simulink model "last_test2"  (Simulink 7.1)
settings: Solver=ode3  StartTime=0.0  StopTime=2000  FixedStep=0.1  RelTol=1e-3
undefined symbols (not defined in the file or in its folder): C_calc, kalmanfilter4
libraries: fordypningsprosjekt x5, marine_gnc x3, simulink x1
settings Model: Creator=anderga  LastModifiedBy=anders
settings OptimizationCC: SimCompilerOptimization=On

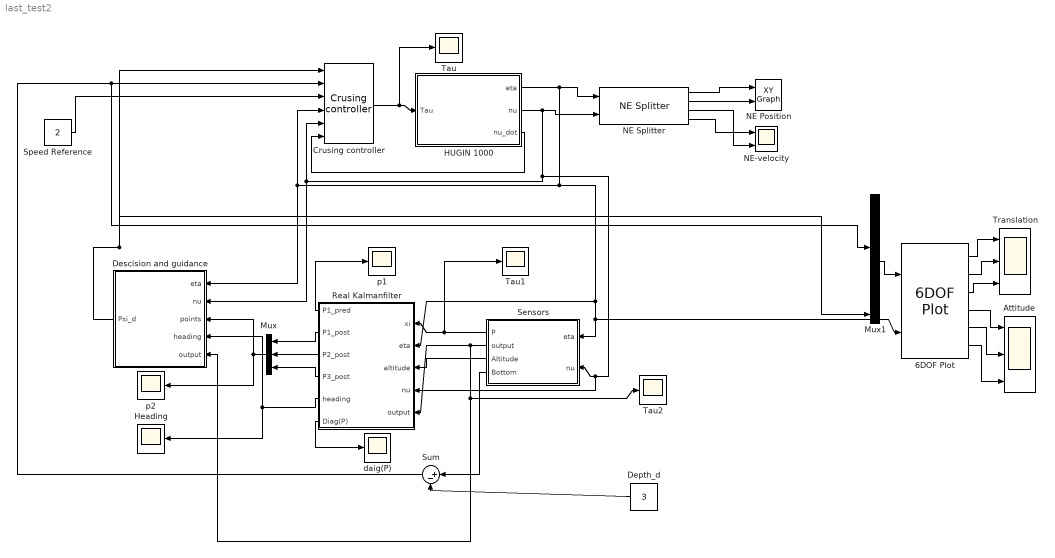
== system last_test2 ==
  6DOF Plot : fordypningsprosjekt/6DOF Plot  SystemSampleTime=-1
  Attitude : Scope  NumInputPorts=3
      settings: TimeRange=700  YMin=-2.5~-10~-50  YMax=2~1~350  SaveName=Attitude
  Crusing controller : fordypningsprosjekt/Crusing controller  SystemSampleTime=-1  Kp_u=10  Ki_u=3  Kp_c=100  Kd_c=100  Kp_d=50  Kp2_d=20  Kd_d=20
  Depth_d : Constant  Orientation=left  Value=3  OutDataType=sfix(16)  OutScaling=2^0
  Descision and guidance : Subsystem  Orientation=left  AncestorBlock=fordypningsprosjekt/Look-ahead guidance
  HUGIN 1000 : Subsystem  AncestorBlock=fordypningsprosjekt/HUGIN 1000  mask(HUGIN 1000 AUV){eta_0=[-30 -30 0 0 0 0], nu_0=[0 0 0 0 0 0], c_on_off=on, beta_c=-45, V_c=0.3}
      mask prompts: eta_0 "Initial Position [x y z phi theta psi]"; nu_0 "Initial speed [u v w p q r]"; c_on_off "Current on"; beta_c "Current heading(deg)"; V_c "Current Velocity"
      mask help:
      | The hydrodynamic model of Kongsberg Maritimes
      | AUV type HUGIN 1000.
      |
      | Implemented using
      |
      | eta_dot = J(eta)*nu
      | M*nu_dot + C(nu)*nu + D(nu)*nu + g(eta) = tau
      |
      | and the MMS toolbox from www.marinecybernetics.org
      mask init:
      | m = 1380;
      | xg = 0;
      | yg = 0;
      | zg = 0.0328;
      | Ix = 86.53;
      | Iy = 1247;
      | Iz = 1247;
      | 
      | Xu = -85.57;
      | Yv = -1092.9;
      | Yr = -84.1448;
      | Zw = -1092.9;
      | Zq = 84.1448;
      | Mq = -795.1686;
      | Nr = -795.1686;
      |     
      | M = [m-Xu   0       0       0       m*zg    -m*yg;
      |      0      m-Yv    0       -m*zg   0       m*xg-Yr;
      |      0      0       m-Zw    m*yg    -m*xg-Zq 0;
      |      0      -m*zg   m*yg    Ix      0        0;
      |      m*zg   0       -m*xg-Zq 0      Iy-Mq    0;
      |      -m*yg  m*xg-Yr 0       0       0       Iz-Nr];
  Heading : Scope
      settings: YMin=1.3258  YMax=1.32584  SaveName=Pipeline_heading
  Mux : Mux  Orientation=left  Inputs=3
  Mux1 : Mux  Inputs=6
  NE Position : simulink/Sinks/XY Graph  SystemSampleTime=-1  xmin=-1000  xmax=1000  ymin=-1000  ymax=1000  st=-1
  NE Splitter : fordypningsprosjekt/NE Splitter  SystemSampleTime=-1
  NE-velocity : Scope  NumInputPorts=2
      settings: YMin=0~-0.25  YMax=2.75~0.2  SaveName=NE_Veloc
  Real Kalmanfilter : Subsystem  Orientation=left  AncestorBlock=fordypningsprosjekt/Real Kalmanfilter
  Sensors : Subsystem  Orientation=left  AncestorBlock=fordypningsprosjekt/Sensors
  Speed Reference : Constant  Value=2  OutDataType=sfix(16)  OutScaling=2^0
  Sum : Sum  Orientation=left  Inputs=|+-  OutDataType=sfix(16)  OutScaling=2^0
  Tau : Scope
      settings: YMin=-3000  YMax=1000  SaveName=Tau_c
  Tau1 : Scope
      settings: TimeRange=700  YMin=-0.5  YMax=0.5  SaveName=Cam_output
  Tau2 : Scope
      settings: TimeRange=700  YMin=0  YMax=1  SaveName=Cam_output1
  Translation : Scope  NumInputPorts=3
      settings: YMin=-150~-200~0  YMax=200~800~12.5  SaveName=Translation
  daig(P) : Scope
      settings: YMin=0  YMax=22.5  SaveName=diag_p_apr
  p1 : Scope
      settings: YMin=0  YMax=500  SaveName=P_pred
  p2 : Scope
      settings: YMin=0  YMax=400  SaveName=P_post
  wires:
  Crusing controller/1 -> HUGIN 1000/1(Tau), Tau/1
  HUGIN 1000/1(eta) -> NE Splitter/1, Real Kalmanfilter/2(eta), Sensors/1(eta), 6DOF Plot/2, Crusing controller/4, Descision and guidance/1(eta)
  HUGIN 1000/2(nu) -> NE Splitter/2, Sensors/2(nu), Real Kalmanfilter/4(nu), Crusing controller/5, Descision and guidance/2(nu)
  NE Splitter/1 -> NE Position/1
  NE Splitter/2 -> NE Position/2
  NE Splitter/4 -> NE-velocity/1
  NE Splitter/3 -> NE-velocity/2
  HUGIN 1000/3(nu_dot) -> Crusing controller/6
  Sensors/1(P) -> Real Kalmanfilter/1(xi), Tau1/1
  Sensors/2(output) -> Descision and guidance/5(output), Tau2/1, Real Kalmanfilter/5(output)
  Sensors/3(Altitude) -> Real Kalmanfilter/3(altitude)
  Depth_d/1 -> Sum/2
  Sensors/4(Bottom) -> Sum/1
  Sum/1 -> Mux1/3, Crusing controller/2
  Speed Reference/1 -> Crusing controller/3
  Descision and guidance/1(Psi_d) -> Mux1/6, Crusing controller/1
  Real Kalmanfilter/5(heading) -> Heading/1, Descision and guidance/4(heading)
  Real Kalmanfilter/2(P1_post) -> Mux/1
  Real Kalmanfilter/3(P2_post) -> Mux/2
  Real Kalmanfilter/4(P3_post) -> Mux/3
  Mux/1 -> p2/1, Descision and guidance/3(points)
  6DOF Plot/1 -> Translation/1
  6DOF Plot/2 -> Translation/2
  6DOF Plot/3 -> Translation/3
  6DOF Plot/4 -> Attitude/1
  6DOF Plot/5 -> Attitude/2
  6DOF Plot/6 -> Attitude/3
  Mux1/1 -> 6DOF Plot/1
  Real Kalmanfilter/1(P1_pred) -> p1/1
  Real Kalmanfilter/6(Diag(P)) -> daig(P)/1

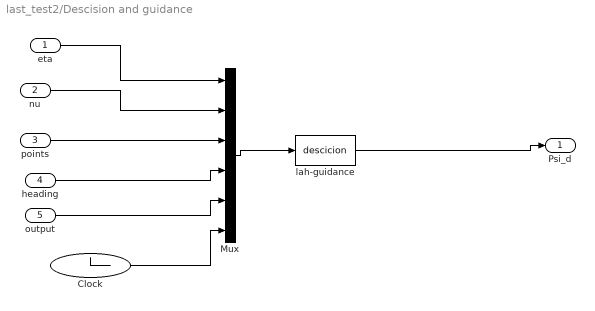
== system last_test2/Descision and guidance ==
  eta : Inport  OutDataType=sfix(16)  OutScaling=2^0
  nu : Inport  Port=2  OutDataType=sfix(16)  OutScaling=2^0
  points : Inport  Port=3  OutDataType=sfix(16)  OutScaling=2^0
  heading : Inport  Port=4  OutDataType=sfix(16)  OutScaling=2^0
  output : Inport  Port=5  OutDataType=sfix(16)  OutScaling=2^0
  Clock : Clock
  Mux : Mux  Inputs=6
  lah-guidance : MATLABFcn  MATLABFcn=descicion  OutputDimensions=1
  Psi_d : Outport  OutDataType=sfix(16)  OutScaling=2^0
  wires:
  heading/1 -> Mux/4
  points/1 -> Mux/3
  eta/1 -> Mux/1
  nu/1 -> Mux/2
  Mux/1 -> lah-guidance/1
  lah-guidance/1 -> Psi_d/1
  output/1 -> Mux/5
  Clock/1 -> Mux/6

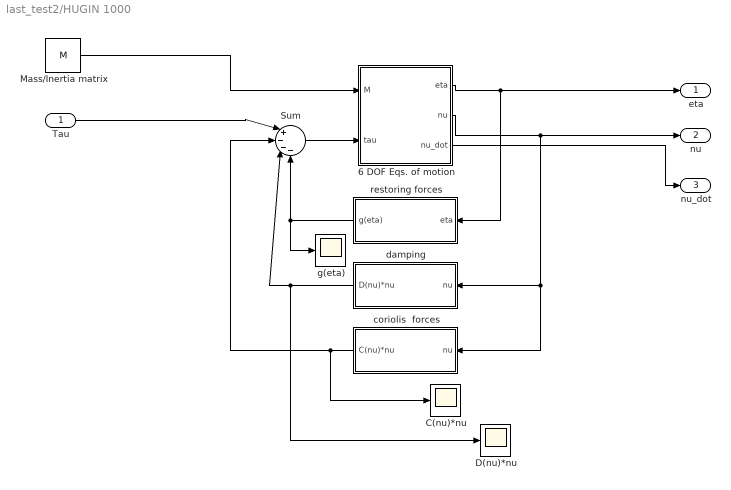
== system last_test2/HUGIN 1000 ==
  Tau : Inport  OutDataType=sfix(16)  OutScaling=2^0
  6 DOF Eqs. of motion : Subsystem  AncestorBlock=marine_gnc/Models/ Kinetics /6 DOF Eqs. of motion  mask(Equations of motion){nu0=nu_0, eta0=eta_0}
      mask prompts: nu0 "Initial velocities (u,v,w,p,q,r)"; eta0 "Initial position/attitude (x,y,z,phi,theta,psi)"
      mask help:
      | 6 DOF equations of motion (surge, sway, heave, roll, pitch and yaw)
      |
      |    eta_dot = J(eta)*nu
      |    (M_RB+M_A)*nu_dot  =  tau
      |
      | where nu = [u,v,w,p,q,r]'  and eta = [x,y,z,phi,theta,psi]'
      |
      | T. I. Fossen (2002). Marine Control Systems: Guidance, Navigation and Control of Ships, Rigs and Underwater Vehicles, Marine Cybernetics AS, ISBN 82-92356-00-2
      |
      | Modified by Anders Garmo (2008)
  C(nu)*nu : Scope
      settings: TimeRange=100  YMin=-0.1  YMax=1.2  SaveName=Coriolis_forces
  D(nu)*nu : Scope
      settings: TimeRange=100  YMin=-10  YMax=100  SaveName=Damping_forces
  Mass/Inertia matrix : Constant  Value=M  OutDataType=sfix(16)  OutScaling=2^0
  Sum : Sum  Inputs=|+---  OutDataType=sfix(16)  OutScaling=2^0
  coriolis  forces : Subsystem  Orientation=left
      mask init:
      | W = 1380*9.81;
      | 
      | zg = 0.0328;
  damping : Subsystem  Orientation=left
      mask init:
      | Xu = -19.1881;
      | Yv = -931.9715;
      | Yr = 1915.8;
      | Zw = -931.9715;
      | Zq = -1915.8;
      | Kp = -1000;
      | Mw = 1760.7;
      | Mq = -8386.3;
      | Nv = -1760.7;
      | Nr = -8386.3;
      | 
      | Xuu = -3.8938;
      | 
      | D = [Xu 0 0 0 0 0;
      |       0 Yv 0 0 0 Yr;
      |       0 0 Zw 0 Zq 0;
      |       0 0 0 Kp 0 0;
      |       0 0 Mw 0 Mq 0;
      |       0 Nv 0 0 0 Nr];
  g(eta) : Scope
      settings: TimeRange=100  YMin=0  YMax=100  SaveName=ScopeData7
  restoring forces : Subsystem  Orientation=left
      mask init:
      | W = 1380*9.81;
      | 
      | zg = 0.0328;
  eta : Outport  OutDataType=sfix(16)  OutScaling=2^0
  nu : Outport  Port=2  OutDataType=sfix(16)  OutScaling=2^0
  nu_dot : Outport  Port=3  OutDataType=sfix(16)  OutScaling=2^0
  wires:
  Mass/Inertia matrix/1 -> 6 DOF Eqs. of motion/1(M)
  6 DOF Eqs. of motion/2(nu) -> nu/1, damping/1(nu), coriolis  forces/1(nu)
  6 DOF Eqs. of motion/1(eta) -> restoring forces/1(eta), eta/1
  Sum/1 -> 6 DOF Eqs. of motion/2(tau)
  Tau/1 -> Sum/1
  coriolis  forces/1(C(nu)*nu) -> C(nu)*nu/1, Sum/2
  restoring forces/1(g(eta)) -> Sum/4, g(eta)/1
  damping/1(D(nu)*nu) -> Sum/3, D(nu)*nu/1
  6 DOF Eqs. of motion/3(nu_dot) -> nu_dot/1

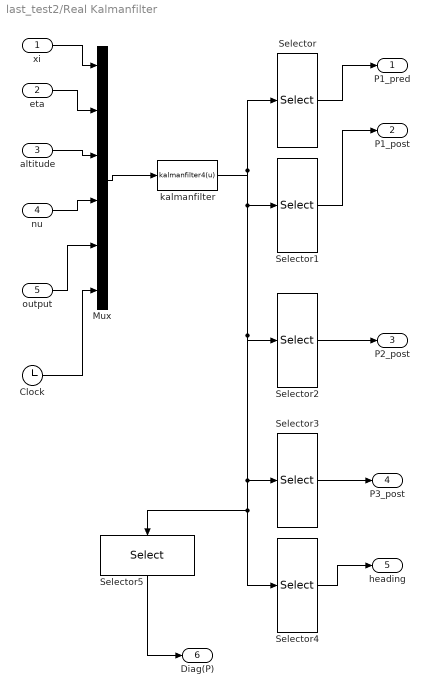
== system last_test2/Real Kalmanfilter ==
  xi : Inport  OutDataType=sfix(16)  OutScaling=2^0
  eta : Inport  Port=2  OutDataType=sfix(16)  OutScaling=2^0
  altitude : Inport  Port=3  OutDataType=sfix(16)  OutScaling=2^0
  nu : Inport  Port=4  OutDataType=sfix(16)  OutScaling=2^0
  output : Inport  Port=5  OutDataType=sfix(16)  OutScaling=2^0
  Clock : Clock
      settings: Decimation=10
  Mux : Mux  Inputs=6
  Selector : Selector  InputPortWidth=17  IndexOptions=Index vector (dialog)  Indices=[1:3]  OutputSizes=1
  Selector1 : Selector  InputPortWidth=17  IndexOptions=Index vector (dialog)  Indices=4:6  OutputSizes=1
  Selector2 : Selector  InputPortWidth=17  IndexOptions=Index vector (dialog)  Indices=7:9  OutputSizes=1
  Selector3 : Selector  InputPortWidth=17  IndexOptions=Index vector (dialog)  Indices=10:12  OutputSizes=1
  Selector4 : Selector  InputPortWidth=17  IndexOptions=Index vector (dialog)  Indices=13  OutputSizes=1
  Selector5 : Selector  Orientation=down  InputPortWidth=17  IndexOptions=Index vector (dialog)  Indices=14:17  OutputSizes=1
  kalmanfilter : MATLABFcn  MATLABFcn=kalmanfilter4(u)  OutputDimensions=17
  P1_pred : Outport  OutDataType=sfix(16)  OutScaling=2^0
  P1_post : Outport  Port=2  OutDataType=sfix(16)  OutScaling=2^0
  P2_post : Outport  Port=3  OutDataType=sfix(16)  OutScaling=2^0
  P3_post : Outport  Port=4  OutDataType=sfix(16)  OutScaling=2^0
  heading : Outport  Port=5  OutDataType=sfix(16)  OutScaling=2^0
  Diag(P) : Outport  Port=6  OutDataType=sfix(16)  OutScaling=2^0
  wires:
  output/1 -> Mux/5
  Mux/1 -> kalmanfilter/1
  nu/1 -> Mux/4
  altitude/1 -> Mux/3
  eta/1 -> Mux/2
  xi/1 -> Mux/1
  kalmanfilter/1 -> Selector/1, Selector1/1, Selector2/1, Selector3/1, Selector4/1, Selector5/1
  Selector/1 -> P1_pred/1
  Selector1/1 -> P1_post/1
  Selector2/1 -> P2_post/1
  Selector3/1 -> P3_post/1
  Selector4/1 -> heading/1
  Clock/1 -> Mux/6
  Selector5/1 -> Diag(P)/1

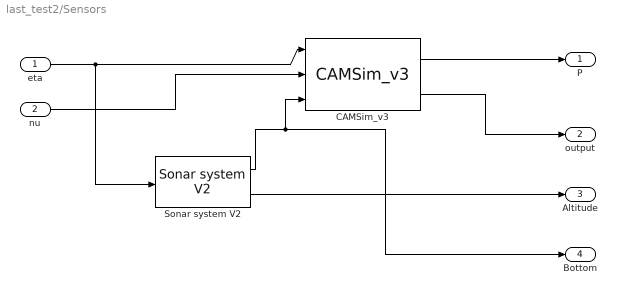
== system last_test2/Sensors ==
  eta : Inport  OutDataType=sfix(16)  OutScaling=2^0
  nu : Inport  Port=2  OutDataType=sfix(16)  OutScaling=2^0
  CAMSim_v3 : fordypningsprosjekt/CAMSim_v3  SystemSampleTime=-1  noise=on  variance=0.01
      link override MATLAB Fcn: MATLABFcn=camsim3
  Sonar system V2 : fordypningsprosjekt/Sonar system V2  SystemSampleTime=-1  sea_bottom=-40
  P : Outport  OutDataType=sfix(16)  OutScaling=2^0
  output : Outport  Port=2  OutDataType=sfix(16)  OutScaling=2^0
  Altitude : Outport  Port=3  OutDataType=sfix(16)  OutScaling=2^0
  Bottom : Outport  Port=4  OutDataType=sfix(16)  OutScaling=2^0
  wires:
  eta/1 -> Sonar system V2/1, CAMSim_v3/1
  nu/1 -> CAMSim_v3/2
  Sonar system V2/1 -> Bottom/1, CAMSim_v3/3
  Sonar system V2/2 -> Altitude/1
  CAMSim_v3/1 -> P/1
  CAMSim_v3/2 -> output/1

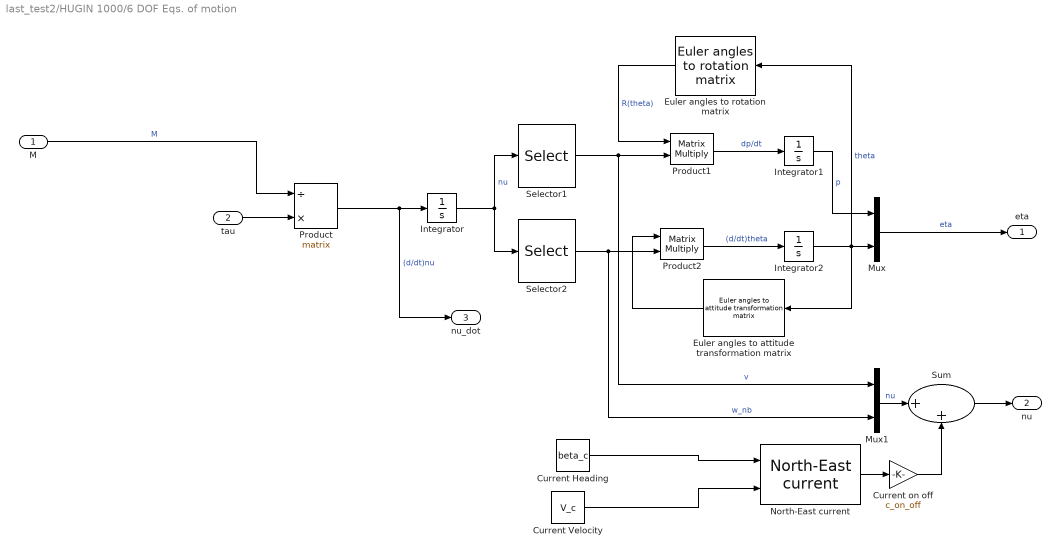
== system last_test2/HUGIN 1000/6 DOF Eqs. of motion ==
  M : Inport  OutDataType=sfix(16)  OutScaling=2^0
  tau : Inport  Port=2  OutDataType=sfix(16)  OutScaling=2^0
  Current Heading : Constant  Value=beta_c  OutDataType=sfix(16)  OutScaling=2^0
  Current Velocity : Constant  Value=V_c  OutDataType=sfix(16)  OutScaling=2^0
  Current on off : Gain  Gain=c_on_off  ParameterDataType=sfix(16)  ParameterScaling=2^0  OutDataType=sfix(16)  OutScaling=2^0
  Euler angles to rotation matrix : marine_gnc/Models/ Kinematics/Euler angles to rotation matrix  Orientation=left  SystemSampleTime=-1
  Euler angles to attitude transformation matrix : marine_gnc/Models/ Kinematics/Euler angles to attitude transformation matrix  Orientation=left  SystemSampleTime=-1
  Integrator : Integrator  InitialCondition=nu0
  Integrator1 : Integrator  InitialCondition=eta0(1:3)
  Integrator2 : Integrator  InitialCondition=eta0(4:6)
  Mux : Mux  Inputs=2
  Mux1 : Mux  Inputs=2
  North-East current : marine_gnc/Environment/Current/North-East current  SystemSampleTime=-1
  Product : Product  Inputs=/*  Multiplication=Matrix(*)  OutDataType=sfix(16)  OutScaling=2^0  SaturateOnIntegerOverflow=on  OutDataTypeStr=Inherit: Same as first input
  Product1 : Product  Inputs=**  Multiplication=Matrix(*)  OutDataType=sfix(16)  OutScaling=2^0  SaturateOnIntegerOverflow=on  OutDataTypeStr=Inherit: Same as first input
  Product2 : Product  Inputs=**  Multiplication=Matrix(*)  OutDataType=sfix(16)  OutScaling=2^0  SaturateOnIntegerOverflow=on  OutDataTypeStr=Inherit: Same as first input
  Selector1 : Selector  InputPortWidth=6  IndexOptions=Index vector (dialog)  Indices=[1 2 3]  OutputSizes=1
  Selector2 : Selector  InputPortWidth=6  IndexOptions=Index vector (dialog)  Indices=[4 5 6]  OutputSizes=1
  Sum : Sum  Inputs=|++  OutDataType=sfix(16)  OutScaling=2^0
  eta : Outport  OutDataType=sfix(16)  OutScaling=2^0
  nu : Outport  Port=2  OutDataType=sfix(16)  OutScaling=2^0
  nu_dot : Outport  Port=3  OutDataType=sfix(16)  OutScaling=2^0
  wires:
  tau/1 -> Product/2
  Euler angles to attitude transformation matrix/1 -> Product2/1
  Mux/1 -> eta/1  "eta"
  Integrator1/1 -> Mux/1  "p"
  Integrator2/1 -> Euler angles to attitude transformation matrix/1, Euler angles to rotation matrix/1, Mux/2  "theta"
  Product2/1 -> Integrator2/1  "(d/dt)theta"
  Euler angles to rotation matrix/1 -> Product1/1  "R(theta)"
  Product1/1 -> Integrator1/1  "dp/dt"
  Selector2/1 -> Product2/2, Mux1/2  "w_nb"
  Selector1/1 -> Mux1/1, Product1/2  "v"
  Integrator/1 -> Selector2/1, Selector1/1  "nu"
  Product/1 -> Integrator/1, nu_dot/1  "(d/dt)nu"
  M/1 -> Product/1  "M"
  Mux1/1 -> Sum/1  "nu"
  Sum/1 -> nu/1
  North-East current/1 -> Current on off/1
  Current Heading/1 -> North-East current/1
  Current Velocity/1 -> North-East current/2
  Current on off/1 -> Sum/2

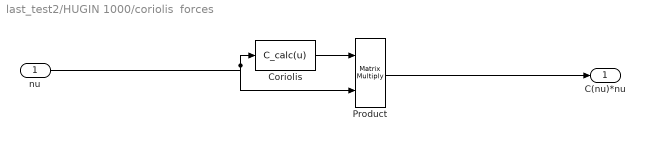
== system last_test2/HUGIN 1000/coriolis  forces ==
  nu : Inport  OutDataType=sfix(16)  OutScaling=2^0
  Coriolis : MATLABFcn  MATLABFcn=C_calc(u)  OutputDimensions=[6,6]  Output1D=off
  Product : Product  Multiplication=Matrix(*)  OutDataType=sfix(16)  OutScaling=2^0  RndMeth=Zero
  C(nu)*nu : Outport  OutDataType=sfix(16)  OutScaling=2^0
  wires:
  nu/1 -> Product/2, Coriolis/1
  Coriolis/1 -> Product/1
  Product/1 -> C(nu)*nu/1

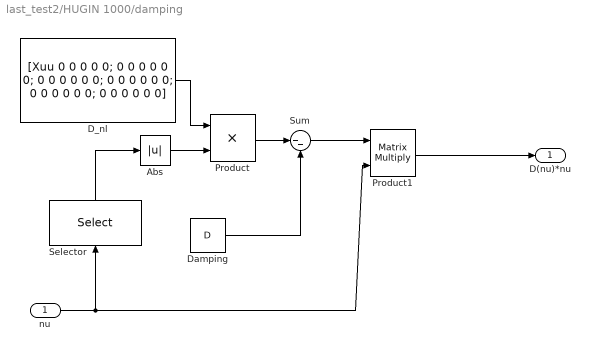
== system last_test2/HUGIN 1000/damping ==
  nu : Inport  OutDataType=sfix(16)  OutScaling=2^0
  Abs : Abs  OutDataType=sfix(16)  OutScaling=2^0
  D_nl : Constant  Value=[Xuu 0 0 0 0 0; 0 0 0 0 0 0; 0 0 0 0 0 0; 0 0 0 0 0 0; 0 0 0 0 0 0; 0 0 0 0 0 0]  OutDataType=sfix(16)  OutScaling=2^0
  Damping : Constant  Value=D  OutDataType=sfix(16)  OutScaling=2^0
  Product : Product  OutDataType=sfix(16)  OutScaling=2^0  RndMeth=Zero
  Product1 : Product  Multiplication=Matrix(*)  OutDataType=sfix(16)  OutScaling=2^0  RndMeth=Zero
  Selector : Selector  Orientation=up  InputPortWidth=6  IndexOptions=Index vector (dialog)  Indices=[1]  OutputSizes=1
  Sum : Sum  Inputs=|--  OutDataType=sfix(16)  OutScaling=2^0
  D(nu)*nu : Outport  OutDataType=sfix(16)  OutScaling=2^0
  wires:
  Damping/1 -> Sum/2
  Product/1 -> Sum/1
  nu/1 -> Product1/2, Selector/1
  D_nl/1 -> Product/1
  Abs/1 -> Product/2
  Sum/1 -> Product1/1
  Product1/1 -> D(nu)*nu/1
  Selector/1 -> Abs/1

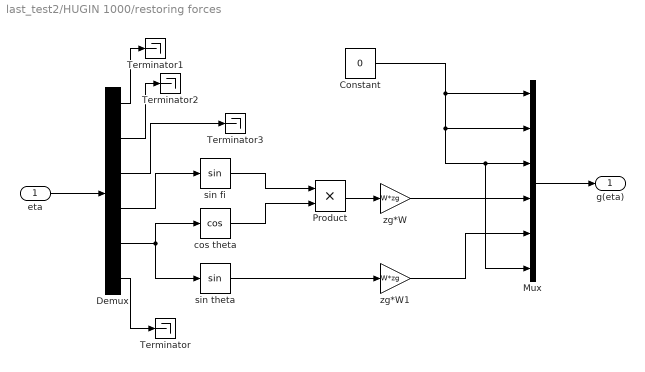
== system last_test2/HUGIN 1000/restoring forces ==
  eta : Inport  OutDataType=sfix(16)  OutScaling=2^0
  Constant : Constant  Value=0  OutDataType=sfix(16)  OutScaling=2^0
  Demux : Demux  Outputs=6
  Mux : Mux  Inputs=6
  Product : Product  OutDataType=sfix(16)  OutScaling=2^0  RndMeth=Zero
  Terminator{,1..3} (4 alike) : Terminator
  cos theta : Trigonometry  Operator=cos
  sin fi : Trigonometry
  sin theta : Trigonometry
  zg*W : Gain  Gain=W*zg  ParameterDataType=sfix(16)  ParameterScaling=2^0  OutDataType=sfix(16)  OutScaling=2^0
  zg*W1 : Gain  Gain=W*zg  ParameterDataType=sfix(16)  ParameterScaling=2^0  OutDataType=sfix(16)  OutScaling=2^0
  g(eta) : Outport  OutDataType=sfix(16)  OutScaling=2^0
  wires:
  eta/1 -> Demux/1
  Demux/4 -> sin fi/1
  Demux/5 -> cos theta/1, sin theta/1
  cos theta/1 -> Product/2
  sin fi/1 -> Product/1
  Product/1 -> zg*W/1
  sin theta/1 -> zg*W1/1
  Mux/1 -> g(eta)/1
  zg*W1/1 -> Mux/5
  zg*W/1 -> Mux/4
  Constant/1 -> Mux/1, Mux/2, Mux/3, Mux/6
  Demux/6 -> Terminator/1
  Demux/1 -> Terminator1/1
  Demux/2 -> Terminator2/1
  Demux/3 -> Terminator3/1
